simulink model "WindFarmType4AverageModel"  (R2024b)
settings: Solver=FixedStepDiscrete  StartTime=0.0  StopTime=5  RelTol=1e-4
PreLoadFcn:
  | Ts=50e-6;
InitFcn:
  | xInitial = WindFarmType4AverageModelInit;
  | Ts=50e-6;
undefined symbols (not defined in the file or in its folder): D1, D11, Delta, DiscIntNeverNeededParam, find_system
libraries: spsSecondOrderFilterLib x54, spsabctodq0Lib x30, spsThreePhaseVIMeasurementLib x26, simulink_extras x24, spsFirstOrderFilterLib x24, spsControlledVoltageSourceLib x18, spsThreePhaseTransformerTwoWindingsLib x14, spsThreePhasePISectionLineLib x14, simulink x12, spsSeriesRLCBranchLib x7, spsThreePhaseSeriesRLCLoadLib x7, spsSynchronousMachinepuStandardLib x7
(part 10 of 14)

== system WindFarmType4AverageModel/Noble Chateaugay (106.5 MW)/Wind Farm/Control/Grid-side converter Control system/INT ==
  note: INTEGRATOR (Trapezoidal) with External limits & Reset & Hold
  Max : Inport
  Min : Inport  Port=2
  In : Inport  Port=3
  Ki : Inport  Port=4
  Hold : Inport  Port=5
  Reset : Inport  Port=6
  Reset Value : Inport  Port=7
  Gain : Gain  Gain=Ts* 0.5  SaturateOnIntegerOverflow=on  OutDataTypeStr=Inherit: Same as input  ParamDataTypeStr=Inherit: Same as input
  IC = 0 : UnitDelay  SampleTime=Ts  HasFrameUpgradeWarning=on
  IC = i_ic : UnitDelay  SampleTime=Ts  HasFrameUpgradeWarning=on
  Logical Operator4 : Logic  Operator=OR
  MinMax : MinMax  Inputs=2  InputSameDT=on  SaturateOnIntegerOverflow=on
  MinMax1 : MinMax  Function=max  Inputs=2  InputSameDT=on  SaturateOnIntegerOverflow=on
  Product : Product  SaturateOnIntegerOverflow=on  OutDataTypeStr=Inherit: Same as first input
  S6 : Subsystem  mask(Limiter with External Limits){}
      mask Display: disp('      Limiter\n')
  Sum : Sum  InputSameDT=on  SaturateOnIntegerOverflow=on  OutDataTypeStr=Inherit: Same as first input
  Sum1 : Sum  InputSameDT=on  SaturateOnIntegerOverflow=on  OutDataTypeStr=Inherit: Same as first input
  Switch2 : Switch  Threshold=0.5
  Switch3 : Switch  Threshold=0.5
  Switch7 : Switch  Threshold=0.5
  Out : Outport  InitialOutput=0  VectorParamsAs1DForOutWhenUnconnected=off
  wires:
  Switch7/1 -> Switch3/1, Sum/2, Switch2/1
  IC = i_ic/1 -> Switch7/3
  Min/1 -> MinMax1/2, Switch3/3
  Switch3/1 -> MinMax1/1
  MinMax1/1 -> S6/3(MIN)
  MinMax/1 -> S6/1(MAX)
  Reset Value/1 -> Switch7/1
  Max/1 -> MinMax/2, Switch2/3
  Switch2/1 -> MinMax/1
  Logical Operator4/1 -> Switch3/2, Switch2/2
  Reset/1 -> Logical Operator4/2, Switch7/2
  Hold/1 -> Logical Operator4/1
  Sum/1 -> S6/2(In)
  Product/1 -> Sum/1
  In/1 -> Sum1/1, IC = 0/1
  IC = 0/1 -> Sum1/2
  Ki/1 -> Gain/1
  Sum1/1 -> Product/2
  Gain/1 -> Product/1
  S6/1("  ") -> Out/1, IC = i_ic/1

== system WindFarmType4AverageModel/Noble Chateaugay (106.5 MW)/Wind Farm/Control/Measurement and Transformation/Discrete 3-phase PLL-Driven Positive-Sequence Active & Reactive Power ==
  note: Pierre Giroux, Gilbert Sybille
      | Power System Simulation Laboratory
      | IREQ, Hydro-Quebc
  note: Discrete 3-phase PLL-driven Positive-Sequence Active & Reactive Power
  Freq : Inport  PortDimensions=1
  w : Inport  Port=2  PortDimensions=1
  Vabc : Inport  Port=3  PortDimensions=3
  Iabc : Inport  Port=4  PortDimensions=3
  Deg->Rad : Gain  Gain=pi/180  SaturateOnIntegerOverflow=on  OutDataTypeStr=Inherit: Same as input  ParamDataTypeStr=Inherit: Same as input
  Discrete 3-phase PLL-Driven Positive-Sequence Fundamental Value : Subsystem  mask(Discrete 3-phase PLL-Driven Positive-Sequence Fundamental Value){Finit=Finit, Fmin=Fmin, Par_Init=Par_Vinit, Ts=Ts}
      mask prompts: Finit "Initial frequency (Hz):"; Fmin "Minimum frequency (Hz):"; Par_Init "Initial input (positive component): [ Mag  Phase-relative-to-PLL(degrees) ]"; Ts "Sample time:"
      mask help:
      | For a supplied fundamental frequency (port Freq), this discrete block computes  the positive-sequence component (Magnitude and Phase)  of a set of three balanced or unbalanced signals (port abc) which may contain harmonics.
      |  Input port "Sin_Cos" (a two-dimension signal) provides the reference frame required for the computation..
      |  First and second outputs return respectively the magnitude and phase (in degrees relative to the PLL phase)) of the fundamental.
      | For the first cycle of simulation, the outputs are held constant to the values specified by the parameter "Initial input".
      | constant to the values specified by the parameter "Initial input". The value of the parameter "Minimum frequency" is used to determine the buffer size of the "Variable Transport Delay" block found inside this subsystem.
      mask init:
      | Real_Init=Par_Init(1)*cos(pi/180*Par_Init(2));
      | Imag_Init=Par_Init(1)*sin(pi/180*Par_Init(2));
      | power_initmask();
      settings: OpenFcn=power_openblockproxy();
  Discrete 3-phase PLL-Driven Positive-Sequence Fundamental Value2 : Subsystem  mask(Discrete 3-phase PLL-Driven Positive-Sequence Fundamental Value){Finit=Finit, Fmin=Fmin, Par_Init=Par_Iinit, Ts=Ts}
      mask prompts: Finit "Initial frequency (Hz):"; Fmin "Minimum frequency (Hz):"; Par_Init "Initial input (positive component): [ Mag  Phase-relative-to-PLL(degrees) ]"; Ts "Sample time:"
      mask help:
      | For a supplied fundamental frequency (port Freq), this discrete block computes  the positive-sequence component (Magnitude and Phase)  of a set of three balanced or unbalanced signals (port abc) which may contain harmonics.
      |  Input port "Sin_Cos" (a two-dimension signal) provides the reference frame required for the computation..
      |  First and second outputs return respectively the magnitude and phase (in degrees relative to the PLL phase)) of the fundamental.
      | For the first cycle of simulation, the outputs are held constant to the values specified by the parameter "Initial input".
      | constant to the values specified by the parameter "Initial input". The value of the parameter "Minimum frequency" is used to determine the buffer size of the "Variable Transport Delay" block found inside this subsystem.
      mask init:
      | Real_Init=Par_Init(1)*cos(pi/180*Par_Init(2));
      | Imag_Init=Par_Init(1)*sin(pi/180*Par_Init(2));
      | power_initmask();
      settings: OpenFcn=power_openblockproxy();
  Gain1 : Gain  Gain=3/2  SaturateOnIntegerOverflow=on  OutDataTypeStr=Inherit: Same as input  ParamDataTypeStr=Inherit: Same as input
  Mux2 : Mux  Inputs=2
  Mux3 : Mux  Inputs=2
  Product : Product  InputSameDT=on  SaturateOnIntegerOverflow=on  OutDataTypeStr=Inherit: Same as first input
  Product1 : Product  InputSameDT=on  SaturateOnIntegerOverflow=on  OutDataTypeStr=Inherit: Same as first input
  Product2 : Product  InputSameDT=on  SaturateOnIntegerOverflow=on  OutDataTypeStr=Inherit: Same as first input
  Sum : Sum  Inputs=+-  InputSameDT=on  SaturateOnIntegerOverflow=on  OutDataTypeStr=Inherit: Same as first input
  Trigonometric Function : Trigonometry
  Trigonometric Function1 : Trigonometry  Operator=cos
  Mag_V_I : Outport  VectorParamsAs1DForOutWhenUnconnected=off
  P_Q : Outport  Port=2  VectorParamsAs1DForOutWhenUnconnected=off
  wires:
  Iabc/1 -> Discrete 3-phase PLL-Driven Positive-Sequence Fundamental Value2/3(abc)
  Discrete 3-phase PLL-Driven Positive-Sequence Fundamental Value2/1(Mag) -> Product2/2, Mux3/2
  Product2/1 -> Product1/2, Product/1
  Gain1/1 -> P_Q/1
  Mux3/1 -> Mag_V_I/1
  Product1/1 -> Mux2/2
  Product/1 -> Mux2/1
  Mux2/1 -> Gain1/1
  Trigonometric Function/1 -> Product1/1
  Trigonometric Function1/1 -> Product/2
  Deg->Rad/1 -> Trigonometric Function/1, Trigonometric Function1/1
  Sum/1 -> Deg->Rad/1
  Discrete 3-phase PLL-Driven Positive-Sequence Fundamental Value2/2(Phase) -> Sum/2
  Discrete 3-phase PLL-Driven Positive-Sequence Fundamental Value/1(Mag) -> Product2/1, Mux3/1
  Discrete 3-phase PLL-Driven Positive-Sequence Fundamental Value/2(Phase) -> Sum/1
  w/1 -> Discrete 3-phase PLL-Driven Positive-Sequence Fundamental Value2/2(w), Discrete 3-phase PLL-Driven Positive-Sequence Fundamental Value/2(w)
  Freq/1 -> Discrete 3-phase PLL-Driven Positive-Sequence Fundamental Value2/1(Freq), Discrete 3-phase PLL-Driven Positive-Sequence Fundamental Value/1(Freq)
  Vabc/1 -> Discrete 3-phase PLL-Driven Positive-Sequence Fundamental Value/3(abc)

== system WindFarmType4AverageModel/Noble Chateaugay (106.5 MW)/Wind Farm/Control/Measurement and Transformation/Filter ==
  Vabc_grid : Inport
  Iabc_grid_conv : Inport  Port=2
  Vabc_LL_s : Inport  Port=3
  Iabc_stator : Inport  Port=4
  IL : Inport  Port=5
  Vdc : Inport  Port=6
  Qref : Inport  Port=7
  wr : Inport  Port=8
  angle_rotor : Inport  Port=9
  Second-Order Filter{,1..6} (7 alike) : spsSecondOrderFilterLib/Second-Order Filter  FilterType=Lowpass  Fo=Freq  Zeta=Zeta  Ts=Ts  Initialize=off  Vac_Init="[0,  0,  60]"  Vdc_Init=0  PlotResponse=off  FreqRange=[0, 500, 1]
  Second-Order Filter7 : spsSecondOrderFilterLib/Second-Order Filter  FilterType=Lowpass  Fo=Freq  Zeta=Zeta  Ts=Ts  Initialize=on  Vac_Init=[0.8 -25 60]*0  Vdc_Init=Vdc_nom  PlotResponse=off  FreqRange=[0, 500, 1]
  Second-Order Filter8 : spsSecondOrderFilterLib/Second-Order Filter  FilterType=Lowpass  Fo=Freq  Zeta=Zeta  Ts=Ts  Initialize=on  Vac_Init=[0.8 -25 60]*0  Vdc_Init=1+init(1)/100  PlotResponse=off  FreqRange=[0, 500, 1]
  "Vabc_grid " : Outport  VectorParamsAs1DForOutWhenUnconnected=off
  "Iabc_grid_conv " : Outport  Port=2  VectorParamsAs1DForOutWhenUnconnected=off
  "Vabc_LL_s " : Outport  Port=3  VectorParamsAs1DForOutWhenUnconnected=off
  "Iabc_stator " : Outport  Port=4  VectorParamsAs1DForOutWhenUnconnected=off
  "IL " : Outport  Port=5  VectorParamsAs1DForOutWhenUnconnected=off
  "Vdc " : Outport  Port=6  VectorParamsAs1DForOutWhenUnconnected=off
  "Qref " : Outport  Port=7  VectorParamsAs1DForOutWhenUnconnected=off
  "wr " : Outport  Port=8  VectorParamsAs1DForOutWhenUnconnected=off
  "angle_rotor " : Outport  Port=9  VectorParamsAs1DForOutWhenUnconnected=off
  wires:
  angle_rotor/1 -> Second-Order Filter6/1
  Second-Order Filter6/1 -> "angle_rotor "/1
  Second-Order Filter/1 -> "Vabc_grid "/1
  Second-Order Filter1/1 -> "Iabc_grid_conv "/1
  Vdc/1 -> Second-Order Filter7/1
  Second-Order Filter7/1 -> "Vdc "/1
  Second-Order Filter3/1 -> "Iabc_stator "/1
  wr/1 -> Second-Order Filter8/1
  Second-Order Filter8/1 -> "wr "/1
  Qref/1 -> Second-Order Filter5/1
  Second-Order Filter5/1 -> "Qref "/1
  IL/1 -> Second-Order Filter4/1
  Second-Order Filter4/1 -> "IL "/1
  Vabc_grid/1 -> Second-Order Filter/1
  Iabc_grid_conv/1 -> Second-Order Filter1/1
  Vabc_LL_s/1 -> Second-Order Filter2/1
  Second-Order Filter2/1 -> "Vabc_LL_s "/1
  Iabc_stator/1 -> Second-Order Filter3/1

== system WindFarmType4AverageModel/Noble Chateaugay (106.5 MW)/Wind Farm/Control/Measurement and Transformation/Stator flux estimator ==
  note: Quasi steady state flux at generator stator
  Vdqs : Inport
  Idqs : Inport  Port=2
  wr : Inport  Port=3
  Divide2 : Product  Inputs=**
  Divide4 : Product  Inputs=*/
  Divide7 : Product  Inputs=**
  Divide8 : Product  Inputs=*/
  First-Order Filter : spsFirstOrderFilterLib/First-Order Filter  FilterType=Lowpass  Tc=Flux_meas_time_constant  Ts=Ts  Initialize=on  Vac_Init=[0, 0, 0]  Vdc_Init=1  PlotResponse=off  FreqRange="[0,  200,  1]"
  Gain : Gain  Gain=-1
  Magnitude of flux : Fcn  Expr=sqrt(u(1)^2+u(2)^2)
  Mux1 : Mux  Inputs=2
  Rs2 : Constant  Value=Resistance
  Rs4 : Constant  Value=Resistance
  Selector1 : Selector  InputPortWidth=2  IndexOptions=Index vector (dialog)  Indices=2  OutputSizes=1
  Selector3 : Selector  InputPortWidth=2  IndexOptions=Index vector (dialog)  Indices=2  OutputSizes=1
  Selector7 : Selector  InputPortWidth=2  IndexOptions=Index vector (dialog)  Indices=1  OutputSizes=1
  Selector8 : Selector  InputPortWidth=2  IndexOptions=Index vector (dialog)  Indices=1  OutputSizes=1
  Sum2 : Sum  Inputs=|+-
  Sum4 : Sum  Inputs=|+-
  avoid division by 0 : Saturate  UpperLimit=inf  LowerLimit=1e-6
  Flux : Outport  VectorParamsAs1DForOutWhenUnconnected=off
  wires:
  First-Order Filter/1 -> Flux/1
  avoid division by 0/1 -> Gain/1, Divide4/2
  Magnitude of flux/1 -> First-Order Filter/1
  Mux1/1 -> Magnitude of flux/1
  Divide8/1 -> Mux1/2  "phi_q"
  Gain/1 -> Divide8/2
  Sum4/1 -> Divide8/1
  Selector8/1 -> Divide7/1  "Id"
  Rs4/1 -> Divide7/2
  Selector7/1 -> Sum4/1  "Vd"
  Divide7/1 -> Sum4/2  "Rs*Id"
  Idqs/1 -> Selector8/1, Selector3/1
  Vdqs/1 -> Selector7/1, Selector1/1
  Selector3/1 -> Divide2/1  "Iq"
  Rs2/1 -> Divide2/2
  Selector1/1 -> Sum2/1  "Vq"
  Divide2/1 -> Sum2/2  "Rs*Iq"
  Divide4/1 -> Mux1/1  "phi_d"
  Sum2/1 -> Divide4/1
  wr/1 -> avoid division by 0/1

== system WindFarmType4AverageModel/Noble Chateaugay (106.5 MW)/Wind Farm/Control/Measurement and Transformation/abc2qd ==
  note: This subsystem converts Vab and Vbc to Vd,Vq. The sine and cosine com-
      | puted here are sent to the inverse transformation subsystem qd/abc.
  Vabc_LL : Inport
  sin_cos : Inport  Port=2
  Fcn2 : Fcn  Expr=(u[4]*(2*u[1]+u[2]) + (sqrt(3)*u[2]*u[3])) * 1/3
  Fcn3 : Fcn  Expr=(u[3]*(2*u[1]+u[2]) + (-sqrt(3)*u[2]*u[4])) * 1/3
  Mux : Mux  Inputs=2
  Mux1 : Mux  Inputs=[ 2 2 ]
  Selector : Selector  InputPortWidth=3  IndexOptions=Index vector (dialog)  Indices=[1 2]  OutputSizes=1
  Vdq : Outport  InitialOutput=0  VectorParamsAs1DForOutWhenUnconnected=off
  wires:
  Fcn3/1 -> Mux/1
  Fcn2/1 -> Mux/2
  Mux1/1 -> Fcn3/1, Fcn2/1
  Vabc_LL/1 -> Selector/1
  sin_cos/1 -> Mux1/2
  Mux/1 -> Vdq/1
  Selector/1 -> Mux1/1

== system WindFarmType4AverageModel/Noble Chateaugay (106.5 MW)/Wind Farm/Control/Speed & Pitch Control/Discrete PI Controller ==
  note: Discrete PID Controller
  note: Pierre Giroux, Gilbert Sybille
      | Power System Simulation Laboratory
      | IREQ, Hydro-Quebc
  Error : Inport  SampleTime=Ts
  Discrete-Time Integrator : DiscreteIntegrator  InitialCondition=Init  SampleTime=Ts  LimitOutput=on  UpperSaturationLimit=UpperLimit  LowerSaturationLimit=LowerLimit  ICPrevOutput=DiscIntNeverNeededParam  ICPrevScaledInput=DiscIntNeverNeededParam
  Kp4 : Gain  Gain=Kp  SaturateOnIntegerOverflow=on  SampleTime=Ts  OutDataTypeStr=Inherit: Same as input  ParamDataTypeStr=Inherit: Same as input
  Kp5 : Gain  Gain=Ki  SaturateOnIntegerOverflow=on  SampleTime=Ts  OutDataTypeStr=Inherit: Same as input  ParamDataTypeStr=Inherit: Same as input
  Saturation2 : Saturate  UpperLimit=UpperLimit  LowerLimit=LowerLimit  SampleTime=Ts
  Sum6 : Sum  InputSameDT=on  SaturateOnIntegerOverflow=on  SampleTime=Ts  OutDataTypeStr=Inherit: Same as first input
  Zero-Order Hold : ZeroOrderHold  SampleTime=Ts
  Out : Outport  SampleTime=Ts  InitialOutput=0  VectorParamsAs1DForOutWhenUnconnected=off
  wires:
  Zero-Order Hold/1 -> Sum6/1
  Saturation2/1 -> Out/1
  Discrete-Time Integrator/1 -> Sum6/2
  Kp4/1 -> Zero-Order Hold/1
  Kp5/1 -> Discrete-Time Integrator/1
  Sum6/1 -> Saturation2/1
  Error/1 -> Kp5/1, Kp4/1

== system WindFarmType4AverageModel/Noble Chateaugay (106.5 MW)/Wind Farm/Control/Speed & Pitch Control/Discrete PI Controller1 ==
  note: Discrete PID Controller
  note: Pierre Giroux, Gilbert Sybille
      | Power System Simulation Laboratory
      | IREQ, Hydro-Quebc
  Error : Inport  SampleTime=Ts
  Discrete-Time Integrator : DiscreteIntegrator  InitialCondition=Init  SampleTime=Ts  LimitOutput=on  UpperSaturationLimit=UpperLimit  LowerSaturationLimit=LowerLimit  ICPrevOutput=DiscIntNeverNeededParam  ICPrevScaledInput=DiscIntNeverNeededParam
  Kp4 : Gain  Gain=Kp  SaturateOnIntegerOverflow=on  SampleTime=Ts  OutDataTypeStr=Inherit: Same as input  ParamDataTypeStr=Inherit: Same as input
  Kp5 : Gain  Gain=Ki  SaturateOnIntegerOverflow=on  SampleTime=Ts  OutDataTypeStr=Inherit: Same as input  ParamDataTypeStr=Inherit: Same as input
  Saturation2 : Saturate  UpperLimit=UpperLimit  LowerLimit=LowerLimit  SampleTime=Ts
  Sum6 : Sum  InputSameDT=on  SaturateOnIntegerOverflow=on  SampleTime=Ts  OutDataTypeStr=Inherit: Same as first input
  Zero-Order Hold : ZeroOrderHold  SampleTime=Ts
  Out : Outport  SampleTime=Ts  InitialOutput=0  VectorParamsAs1DForOutWhenUnconnected=off
  wires:
  Zero-Order Hold/1 -> Sum6/1
  Saturation2/1 -> Out/1
  Discrete-Time Integrator/1 -> Sum6/2
  Kp4/1 -> Zero-Order Hold/1
  Kp5/1 -> Discrete-Time Integrator/1
  Sum6/1 -> Saturation2/1
  Error/1 -> Kp5/1, Kp4/1

== system WindFarmType4AverageModel/Noble Chateaugay (106.5 MW)/Wind Farm/Control/Speed & Pitch Control/Discrete PI Controller2 ==
  note: Discrete PID Controller
  note: Pierre Giroux, Gilbert Sybille
      | Power System Simulation Laboratory
      | IREQ, Hydro-Quebc
  Error : Inport  SampleTime=Ts
  Discrete-Time Integrator : DiscreteIntegrator  InitialCondition=Init  SampleTime=Ts  LimitOutput=on  UpperSaturationLimit=UpperLimit  LowerSaturationLimit=LowerLimit  ICPrevOutput=DiscIntNeverNeededParam  ICPrevScaledInput=DiscIntNeverNeededParam
  Kp4 : Gain  Gain=Kp  SaturateOnIntegerOverflow=on  SampleTime=Ts  OutDataTypeStr=Inherit: Same as input  ParamDataTypeStr=Inherit: Same as input
  Kp5 : Gain  Gain=Ki  SaturateOnIntegerOverflow=on  SampleTime=Ts  OutDataTypeStr=Inherit: Same as input  ParamDataTypeStr=Inherit: Same as input
  Saturation2 : Saturate  UpperLimit=UpperLimit  LowerLimit=LowerLimit  SampleTime=Ts
  Sum6 : Sum  InputSameDT=on  SaturateOnIntegerOverflow=on  SampleTime=Ts  OutDataTypeStr=Inherit: Same as first input
  Zero-Order Hold : ZeroOrderHold  SampleTime=Ts
  Out : Outport  SampleTime=Ts  InitialOutput=0  VectorParamsAs1DForOutWhenUnconnected=off
  wires:
  Zero-Order Hold/1 -> Sum6/1
  Saturation2/1 -> Out/1
  Discrete-Time Integrator/1 -> Sum6/2
  Kp4/1 -> Zero-Order Hold/1
  Kp5/1 -> Discrete-Time Integrator/1
  Sum6/1 -> Saturation2/1
  Error/1 -> Kp5/1, Kp4/1

== system WindFarmType4AverageModel/Noble Clinton (100.5 MW)/Wind Farm/Control/Excitation Control system/Discrete PI Controller ==
  note: Discrete PID Controller
  note: Pierre Giroux, Gilbert Sybille
      | Power System Simulation Laboratory
      | IREQ, Hydro-Quebc
  Error : Inport  SampleTime=Ts
  Discrete-Time Integrator : DiscreteIntegrator  InitialCondition=Init  SampleTime=Ts  LimitOutput=on  UpperSaturationLimit=UpperLimit  LowerSaturationLimit=LowerLimit  ICPrevOutput=DiscIntNeverNeededParam  ICPrevScaledInput=DiscIntNeverNeededParam
  Kp4 : Gain  Gain=Kp  SaturateOnIntegerOverflow=on  SampleTime=Ts  OutDataTypeStr=Inherit: Same as input  ParamDataTypeStr=Inherit: Same as input
  Kp5 : Gain  Gain=Ki  SaturateOnIntegerOverflow=on  SampleTime=Ts  OutDataTypeStr=Inherit: Same as input  ParamDataTypeStr=Inherit: Same as input
  Saturation2 : Saturate  UpperLimit=UpperLimit  LowerLimit=LowerLimit  SampleTime=Ts
  Sum6 : Sum  InputSameDT=on  SaturateOnIntegerOverflow=on  SampleTime=Ts  OutDataTypeStr=Inherit: Same as first input
  Zero-Order Hold : ZeroOrderHold  SampleTime=Ts
  Out : Outport  SampleTime=Ts  InitialOutput=0  VectorParamsAs1DForOutWhenUnconnected=off
  wires:
  Zero-Order Hold/1 -> Sum6/1
  Saturation2/1 -> Out/1
  Discrete-Time Integrator/1 -> Sum6/2
  Kp4/1 -> Zero-Order Hold/1
  Kp5/1 -> Discrete-Time Integrator/1
  Sum6/1 -> Saturation2/1
  Error/1 -> Kp5/1, Kp4/1

== system WindFarmType4AverageModel/Noble Clinton (100.5 MW)/Wind Farm/Control/Grid-side converter Control system/Discrete PI Controller ==
  note: Discrete PID Controller
  note: Pierre Giroux, Gilbert Sybille
      | Power System Simulation Laboratory
      | IREQ, Hydro-Quebc
  Error : Inport  SampleTime=Ts
  Discrete-Time Integrator : DiscreteIntegrator  InitialCondition=Init  SampleTime=Ts  LimitOutput=on  UpperSaturationLimit=UpperLimit  LowerSaturationLimit=LowerLimit  ICPrevOutput=DiscIntNeverNeededParam  ICPrevScaledInput=DiscIntNeverNeededParam
  Kp4 : Gain  Gain=Kp  SaturateOnIntegerOverflow=on  SampleTime=Ts  OutDataTypeStr=Inherit: Same as input  ParamDataTypeStr=Inherit: Same as input
  Kp5 : Gain  Gain=Ki  SaturateOnIntegerOverflow=on  SampleTime=Ts  OutDataTypeStr=Inherit: Same as input  ParamDataTypeStr=Inherit: Same as input
  Saturation2 : Saturate  UpperLimit=UpperLimit  LowerLimit=LowerLimit  SampleTime=Ts
  Sum6 : Sum  InputSameDT=on  SaturateOnIntegerOverflow=on  SampleTime=Ts  OutDataTypeStr=Inherit: Same as first input
  Zero-Order Hold : ZeroOrderHold  SampleTime=Ts
  Out : Outport  SampleTime=Ts  InitialOutput=0  VectorParamsAs1DForOutWhenUnconnected=off
  wires:
  Zero-Order Hold/1 -> Sum6/1
  Saturation2/1 -> Out/1
  Discrete-Time Integrator/1 -> Sum6/2
  Kp4/1 -> Zero-Order Hold/1
  Kp5/1 -> Discrete-Time Integrator/1
  Sum6/1 -> Saturation2/1
  Error/1 -> Kp5/1, Kp4/1

== system WindFarmType4AverageModel/Noble Clinton (100.5 MW)/Wind Farm/Control/Grid-side converter Control system/Discrete PI Controller1 ==
  note: Discrete PID Controller
  note: Pierre Giroux, Gilbert Sybille
      | Power System Simulation Laboratory
      | IREQ, Hydro-Quebc
  Error : Inport  SampleTime=Ts
  Discrete-Time Integrator : DiscreteIntegrator  InitialCondition=Init  SampleTime=Ts  LimitOutput=on  UpperSaturationLimit=UpperLimit  LowerSaturationLimit=LowerLimit  ICPrevOutput=DiscIntNeverNeededParam  ICPrevScaledInput=DiscIntNeverNeededParam
  Kp4 : Gain  Gain=Kp  SaturateOnIntegerOverflow=on  SampleTime=Ts  OutDataTypeStr=Inherit: Same as input  ParamDataTypeStr=Inherit: Same as input
  Kp5 : Gain  Gain=Ki  SaturateOnIntegerOverflow=on  SampleTime=Ts  OutDataTypeStr=Inherit: Same as input  ParamDataTypeStr=Inherit: Same as input
  Saturation2 : Saturate  UpperLimit=UpperLimit  LowerLimit=LowerLimit  SampleTime=Ts
  Sum6 : Sum  InputSameDT=on  SaturateOnIntegerOverflow=on  SampleTime=Ts  OutDataTypeStr=Inherit: Same as first input
  Zero-Order Hold : ZeroOrderHold  SampleTime=Ts
  Out : Outport  SampleTime=Ts  InitialOutput=0  VectorParamsAs1DForOutWhenUnconnected=off
  wires:
  Zero-Order Hold/1 -> Sum6/1
  Saturation2/1 -> Out/1
  Discrete-Time Integrator/1 -> Sum6/2
  Kp4/1 -> Zero-Order Hold/1
  Kp5/1 -> Discrete-Time Integrator/1
  Sum6/1 -> Saturation2/1
  Error/1 -> Kp5/1, Kp4/1

== system WindFarmType4AverageModel/Noble Clinton (100.5 MW)/Wind Farm/Control/Grid-side converter Control system/INT ==
  note: INTEGRATOR (Trapezoidal) with External limits & Reset & Hold
  Max : Inport
  Min : Inport  Port=2
  In : Inport  Port=3
  Ki : Inport  Port=4
  Hold : Inport  Port=5
  Reset : Inport  Port=6
  Reset Value : Inport  Port=7
  Gain : Gain  Gain=Ts* 0.5  SaturateOnIntegerOverflow=on  OutDataTypeStr=Inherit: Same as input  ParamDataTypeStr=Inherit: Same as input
  IC = 0 : UnitDelay  SampleTime=Ts  HasFrameUpgradeWarning=on
  IC = i_ic : UnitDelay  SampleTime=Ts  HasFrameUpgradeWarning=on
  Logical Operator4 : Logic  Operator=OR
  MinMax : MinMax  Inputs=2  InputSameDT=on  SaturateOnIntegerOverflow=on
  MinMax1 : MinMax  Function=max  Inputs=2  InputSameDT=on  SaturateOnIntegerOverflow=on
  Product : Product  SaturateOnIntegerOverflow=on  OutDataTypeStr=Inherit: Same as first input
  S6 : Subsystem  mask(Limiter with External Limits){}
      mask Display: disp('      Limiter\n')
  Sum : Sum  InputSameDT=on  SaturateOnIntegerOverflow=on  OutDataTypeStr=Inherit: Same as first input
  Sum1 : Sum  InputSameDT=on  SaturateOnIntegerOverflow=on  OutDataTypeStr=Inherit: Same as first input
  Switch2 : Switch  Threshold=0.5
  Switch3 : Switch  Threshold=0.5
  Switch7 : Switch  Threshold=0.5
  Out : Outport  InitialOutput=0  VectorParamsAs1DForOutWhenUnconnected=off
  wires:
  Switch7/1 -> Switch3/1, Sum/2, Switch2/1
  IC = i_ic/1 -> Switch7/3
  Min/1 -> MinMax1/2, Switch3/3
  Switch3/1 -> MinMax1/1
  MinMax1/1 -> S6/3(MIN)
  MinMax/1 -> S6/1(MAX)
  Reset Value/1 -> Switch7/1
  Max/1 -> MinMax/2, Switch2/3
  Switch2/1 -> MinMax/1
  Logical Operator4/1 -> Switch3/2, Switch2/2
  Reset/1 -> Logical Operator4/2, Switch7/2
  Hold/1 -> Logical Operator4/1
  Sum/1 -> S6/2(In)
  Product/1 -> Sum/1
  In/1 -> Sum1/1, IC = 0/1
  IC = 0/1 -> Sum1/2
  Ki/1 -> Gain/1
  Sum1/1 -> Product/2
  Gain/1 -> Product/1
  S6/1("  ") -> Out/1, IC = i_ic/1

== system WindFarmType4AverageModel/Noble Clinton (100.5 MW)/Wind Farm/Control/Measurement and Transformation/Discrete 3-phase PLL-Driven Positive-Sequence Active & Reactive Power ==
  note: Pierre Giroux, Gilbert Sybille
      | Power System Simulation Laboratory
      | IREQ, Hydro-Quebc
  note: Discrete 3-phase PLL-driven Positive-Sequence Active & Reactive Power
  Freq : Inport  PortDimensions=1
  w : Inport  Port=2  PortDimensions=1
  Vabc : Inport  Port=3  PortDimensions=3
  Iabc : Inport  Port=4  PortDimensions=3
  Deg->Rad : Gain  Gain=pi/180  SaturateOnIntegerOverflow=on  OutDataTypeStr=Inherit: Same as input  ParamDataTypeStr=Inherit: Same as input
  Discrete 3-phase PLL-Driven Positive-Sequence Fundamental Value : Subsystem  mask(Discrete 3-phase PLL-Driven Positive-Sequence Fundamental Value){Finit=Finit, Fmin=Fmin, Par_Init=Par_Vinit, Ts=Ts}
      mask prompts: Finit "Initial frequency (Hz):"; Fmin "Minimum frequency (Hz):"; Par_Init "Initial input (positive component): [ Mag  Phase-relative-to-PLL(degrees) ]"; Ts "Sample time:"
      mask help:
      | For a supplied fundamental frequency (port Freq), this discrete block computes  the positive-sequence component (Magnitude and Phase)  of a set of three balanced or unbalanced signals (port abc) which may contain harmonics.
      |  Input port "Sin_Cos" (a two-dimension signal) provides the reference frame required for the computation..
      |  First and second outputs return respectively the magnitude and phase (in degrees relative to the PLL phase)) of the fundamental.
      | For the first cycle of simulation, the outputs are held constant to the values specified by the parameter "Initial input".
      | constant to the values specified by the parameter "Initial input". The value of the parameter "Minimum frequency" is used to determine the buffer size of the "Variable Transport Delay" block found inside this subsystem.
      mask init:
      | Real_Init=Par_Init(1)*cos(pi/180*Par_Init(2));
      | Imag_Init=Par_Init(1)*sin(pi/180*Par_Init(2));
      | power_initmask();
      settings: OpenFcn=power_openblockproxy();
  Discrete 3-phase PLL-Driven Positive-Sequence Fundamental Value2 : Subsystem  mask(Discrete 3-phase PLL-Driven Positive-Sequence Fundamental Value){Finit=Finit, Fmin=Fmin, Par_Init=Par_Iinit, Ts=Ts}
      mask prompts: Finit "Initial frequency (Hz):"; Fmin "Minimum frequency (Hz):"; Par_Init "Initial input (positive component): [ Mag  Phase-relative-to-PLL(degrees) ]"; Ts "Sample time:"
      mask help:
      | For a supplied fundamental frequency (port Freq), this discrete block computes  the positive-sequence component (Magnitude and Phase)  of a set of three balanced or unbalanced signals (port abc) which may contain harmonics.
      |  Input port "Sin_Cos" (a two-dimension signal) provides the reference frame required for the computation..
      |  First and second outputs return respectively the magnitude and phase (in degrees relative to the PLL phase)) of the fundamental.
      | For the first cycle of simulation, the outputs are held constant to the values specified by the parameter "Initial input".
      | constant to the values specified by the parameter "Initial input". The value of the parameter "Minimum frequency" is used to determine the buffer size of the "Variable Transport Delay" block found inside this subsystem.
      mask init:
      | Real_Init=Par_Init(1)*cos(pi/180*Par_Init(2));
      | Imag_Init=Par_Init(1)*sin(pi/180*Par_Init(2));
      | power_initmask();
      settings: OpenFcn=power_openblockproxy();
  Gain1 : Gain  Gain=3/2  SaturateOnIntegerOverflow=on  OutDataTypeStr=Inherit: Same as input  ParamDataTypeStr=Inherit: Same as input
  Mux2 : Mux  Inputs=2
  Mux3 : Mux  Inputs=2
  Product : Product  InputSameDT=on  SaturateOnIntegerOverflow=on  OutDataTypeStr=Inherit: Same as first input
  Product1 : Product  InputSameDT=on  SaturateOnIntegerOverflow=on  OutDataTypeStr=Inherit: Same as first input
  Product2 : Product  InputSameDT=on  SaturateOnIntegerOverflow=on  OutDataTypeStr=Inherit: Same as first input
  Sum : Sum  Inputs=+-  InputSameDT=on  SaturateOnIntegerOverflow=on  OutDataTypeStr=Inherit: Same as first input
  Trigonometric Function : Trigonometry
  Trigonometric Function1 : Trigonometry  Operator=cos
  Mag_V_I : Outport  VectorParamsAs1DForOutWhenUnconnected=off
  P_Q : Outport  Port=2  VectorParamsAs1DForOutWhenUnconnected=off
  wires:
  Iabc/1 -> Discrete 3-phase PLL-Driven Positive-Sequence Fundamental Value2/3(abc)
  Discrete 3-phase PLL-Driven Positive-Sequence Fundamental Value2/1(Mag) -> Product2/2, Mux3/2
  Product2/1 -> Product1/2, Product/1
  Gain1/1 -> P_Q/1
  Mux3/1 -> Mag_V_I/1
  Product1/1 -> Mux2/2
  Product/1 -> Mux2/1
  Mux2/1 -> Gain1/1
  Trigonometric Function/1 -> Product1/1
  Trigonometric Function1/1 -> Product/2
  Deg->Rad/1 -> Trigonometric Function/1, Trigonometric Function1/1
  Sum/1 -> Deg->Rad/1
  Discrete 3-phase PLL-Driven Positive-Sequence Fundamental Value2/2(Phase) -> Sum/2
  Discrete 3-phase PLL-Driven Positive-Sequence Fundamental Value/1(Mag) -> Product2/1, Mux3/1
  Discrete 3-phase PLL-Driven Positive-Sequence Fundamental Value/2(Phase) -> Sum/1
  w/1 -> Discrete 3-phase PLL-Driven Positive-Sequence Fundamental Value2/2(w), Discrete 3-phase PLL-Driven Positive-Sequence Fundamental Value/2(w)
  Freq/1 -> Discrete 3-phase PLL-Driven Positive-Sequence Fundamental Value2/1(Freq), Discrete 3-phase PLL-Driven Positive-Sequence Fundamental Value/1(Freq)
  Vabc/1 -> Discrete 3-phase PLL-Driven Positive-Sequence Fundamental Value/3(abc)

== system WindFarmType4AverageModel/Noble Clinton (100.5 MW)/Wind Farm/Control/Measurement and Transformation/Filter ==
  Vabc_grid : Inport
  Iabc_grid_conv : Inport  Port=2
  Vabc_LL_s : Inport  Port=3
  Iabc_stator : Inport  Port=4
  IL : Inport  Port=5
  Vdc : Inport  Port=6
  Qref : Inport  Port=7
  wr : Inport  Port=8
  angle_rotor : Inport  Port=9
  Second-Order Filter{,1..6} (7 alike) : spsSecondOrderFilterLib/Second-Order Filter  FilterType=Lowpass  Fo=Freq  Zeta=Zeta  Ts=Ts  Initialize=off  Vac_Init="[0,  0,  60]"  Vdc_Init=0  PlotResponse=off  FreqRange=[0, 500, 1]
  Second-Order Filter7 : spsSecondOrderFilterLib/Second-Order Filter  FilterType=Lowpass  Fo=Freq  Zeta=Zeta  Ts=Ts  Initialize=on  Vac_Init=[0.8 -25 60]*0  Vdc_Init=Vdc_nom  PlotResponse=off  FreqRange=[0, 500, 1]
  Second-Order Filter8 : spsSecondOrderFilterLib/Second-Order Filter  FilterType=Lowpass  Fo=Freq  Zeta=Zeta  Ts=Ts  Initialize=on  Vac_Init=[0.8 -25 60]*0  Vdc_Init=1+init(1)/100  PlotResponse=off  FreqRange=[0, 500, 1]
  "Vabc_grid " : Outport  VectorParamsAs1DForOutWhenUnconnected=off
  "Iabc_grid_conv " : Outport  Port=2  VectorParamsAs1DForOutWhenUnconnected=off
  "Vabc_LL_s " : Outport  Port=3  VectorParamsAs1DForOutWhenUnconnected=off
  "Iabc_stator " : Outport  Port=4  VectorParamsAs1DForOutWhenUnconnected=off
  "IL " : Outport  Port=5  VectorParamsAs1DForOutWhenUnconnected=off
  "Vdc " : Outport  Port=6  VectorParamsAs1DForOutWhenUnconnected=off
  "Qref " : Outport  Port=7  VectorParamsAs1DForOutWhenUnconnected=off
  "wr " : Outport  Port=8  VectorParamsAs1DForOutWhenUnconnected=off
  "angle_rotor " : Outport  Port=9  VectorParamsAs1DForOutWhenUnconnected=off
  wires:
  angle_rotor/1 -> Second-Order Filter6/1
  Second-Order Filter6/1 -> "angle_rotor "/1
  Second-Order Filter/1 -> "Vabc_grid "/1
  Second-Order Filter1/1 -> "Iabc_grid_conv "/1
  Vdc/1 -> Second-Order Filter7/1
  Second-Order Filter7/1 -> "Vdc "/1
  Second-Order Filter3/1 -> "Iabc_stator "/1
  wr/1 -> Second-Order Filter8/1
  Second-Order Filter8/1 -> "wr "/1
  Qref/1 -> Second-Order Filter5/1
  Second-Order Filter5/1 -> "Qref "/1
  IL/1 -> Second-Order Filter4/1
  Second-Order Filter4/1 -> "IL "/1
  Vabc_grid/1 -> Second-Order Filter/1
  Iabc_grid_conv/1 -> Second-Order Filter1/1
  Vabc_LL_s/1 -> Second-Order Filter2/1
  Second-Order Filter2/1 -> "Vabc_LL_s "/1
  Iabc_stator/1 -> Second-Order Filter3/1

== system WindFarmType4AverageModel/Noble Clinton (100.5 MW)/Wind Farm/Control/Measurement and Transformation/Stator flux estimator ==
  note: Quasi steady state flux at generator stator
  Vdqs : Inport
  Idqs : Inport  Port=2
  wr : Inport  Port=3
  Divide2 : Product  Inputs=**
  Divide4 : Product  Inputs=*/
  Divide7 : Product  Inputs=**
  Divide8 : Product  Inputs=*/
  First-Order Filter : spsFirstOrderFilterLib/First-Order Filter  FilterType=Lowpass  Tc=Flux_meas_time_constant  Ts=Ts  Initialize=on  Vac_Init=[0, 0, 0]  Vdc_Init=1  PlotResponse=off  FreqRange="[0,  200,  1]"
  Gain : Gain  Gain=-1
  Magnitude of flux : Fcn  Expr=sqrt(u(1)^2+u(2)^2)
  Mux1 : Mux  Inputs=2
  Rs2 : Constant  Value=Resistance
  Rs4 : Constant  Value=Resistance
  Selector1 : Selector  InputPortWidth=2  IndexOptions=Index vector (dialog)  Indices=2  OutputSizes=1
  Selector3 : Selector  InputPortWidth=2  IndexOptions=Index vector (dialog)  Indices=2  OutputSizes=1
  Selector7 : Selector  InputPortWidth=2  IndexOptions=Index vector (dialog)  Indices=1  OutputSizes=1
  Selector8 : Selector  InputPortWidth=2  IndexOptions=Index vector (dialog)  Indices=1  OutputSizes=1
  Sum2 : Sum  Inputs=|+-
  Sum4 : Sum  Inputs=|+-
  avoid division by 0 : Saturate  UpperLimit=inf  LowerLimit=1e-6
  Flux : Outport  VectorParamsAs1DForOutWhenUnconnected=off
  wires:
  First-Order Filter/1 -> Flux/1
  avoid division by 0/1 -> Gain/1, Divide4/2
  Magnitude of flux/1 -> First-Order Filter/1
  Mux1/1 -> Magnitude of flux/1
  Divide8/1 -> Mux1/2  "phi_q"
  Gain/1 -> Divide8/2
  Sum4/1 -> Divide8/1
  Selector8/1 -> Divide7/1  "Id"
  Rs4/1 -> Divide7/2
  Selector7/1 -> Sum4/1  "Vd"
  Divide7/1 -> Sum4/2  "Rs*Id"
  Idqs/1 -> Selector8/1, Selector3/1
  Vdqs/1 -> Selector7/1, Selector1/1
  Selector3/1 -> Divide2/1  "Iq"
  Rs2/1 -> Divide2/2
  Selector1/1 -> Sum2/1  "Vq"
  Divide2/1 -> Sum2/2  "Rs*Iq"
  Divide4/1 -> Mux1/1  "phi_d"
  Sum2/1 -> Divide4/1
  wr/1 -> avoid division by 0/1

== system WindFarmType4AverageModel/Noble Clinton (100.5 MW)/Wind Farm/Control/Measurement and Transformation/abc2qd ==
  note: This subsystem converts Vab and Vbc to Vd,Vq. The sine and cosine com-
      | puted here are sent to the inverse transformation subsystem qd/abc.
  Vabc_LL : Inport
  sin_cos : Inport  Port=2
  Fcn2 : Fcn  Expr=(u[4]*(2*u[1]+u[2]) + (sqrt(3)*u[2]*u[3])) * 1/3
  Fcn3 : Fcn  Expr=(u[3]*(2*u[1]+u[2]) + (-sqrt(3)*u[2]*u[4])) * 1/3
  Mux : Mux  Inputs=2
  Mux1 : Mux  Inputs=[ 2 2 ]
  Selector : Selector  InputPortWidth=3  IndexOptions=Index vector (dialog)  Indices=[1 2]  OutputSizes=1
  Vdq : Outport  InitialOutput=0  VectorParamsAs1DForOutWhenUnconnected=off
  wires:
  Fcn3/1 -> Mux/1
  Fcn2/1 -> Mux/2
  Mux1/1 -> Fcn3/1, Fcn2/1
  Vabc_LL/1 -> Selector/1
  sin_cos/1 -> Mux1/2
  Mux/1 -> Vdq/1
  Selector/1 -> Mux1/1

== system WindFarmType4AverageModel/Noble Clinton (100.5 MW)/Wind Farm/Control/Speed & Pitch Control/Discrete PI Controller ==
  note: Discrete PID Controller
  note: Pierre Giroux, Gilbert Sybille
      | Power System Simulation Laboratory
      | IREQ, Hydro-Quebc
  Error : Inport  SampleTime=Ts
  Discrete-Time Integrator : DiscreteIntegrator  InitialCondition=Init  SampleTime=Ts  LimitOutput=on  UpperSaturationLimit=UpperLimit  LowerSaturationLimit=LowerLimit  ICPrevOutput=DiscIntNeverNeededParam  ICPrevScaledInput=DiscIntNeverNeededParam
  Kp4 : Gain  Gain=Kp  SaturateOnIntegerOverflow=on  SampleTime=Ts  OutDataTypeStr=Inherit: Same as input  ParamDataTypeStr=Inherit: Same as input
  Kp5 : Gain  Gain=Ki  SaturateOnIntegerOverflow=on  SampleTime=Ts  OutDataTypeStr=Inherit: Same as input  ParamDataTypeStr=Inherit: Same as input
  Saturation2 : Saturate  UpperLimit=UpperLimit  LowerLimit=LowerLimit  SampleTime=Ts
  Sum6 : Sum  InputSameDT=on  SaturateOnIntegerOverflow=on  SampleTime=Ts  OutDataTypeStr=Inherit: Same as first input
  Zero-Order Hold : ZeroOrderHold  SampleTime=Ts
  Out : Outport  SampleTime=Ts  InitialOutput=0  VectorParamsAs1DForOutWhenUnconnected=off
  wires:
  Zero-Order Hold/1 -> Sum6/1
  Saturation2/1 -> Out/1
  Discrete-Time Integrator/1 -> Sum6/2
  Kp4/1 -> Zero-Order Hold/1
  Kp5/1 -> Discrete-Time Integrator/1
  Sum6/1 -> Saturation2/1
  Error/1 -> Kp5/1, Kp4/1

== system WindFarmType4AverageModel/Noble Clinton (100.5 MW)/Wind Farm/Control/Speed & Pitch Control/Discrete PI Controller1 ==
  note: Discrete PID Controller
  note: Pierre Giroux, Gilbert Sybille
      | Power System Simulation Laboratory
      | IREQ, Hydro-Quebc
  Error : Inport  SampleTime=Ts
  Discrete-Time Integrator : DiscreteIntegrator  InitialCondition=Init  SampleTime=Ts  LimitOutput=on  UpperSaturationLimit=UpperLimit  LowerSaturationLimit=LowerLimit  ICPrevOutput=DiscIntNeverNeededParam  ICPrevScaledInput=DiscIntNeverNeededParam
  Kp4 : Gain  Gain=Kp  SaturateOnIntegerOverflow=on  SampleTime=Ts  OutDataTypeStr=Inherit: Same as input  ParamDataTypeStr=Inherit: Same as input
  Kp5 : Gain  Gain=Ki  SaturateOnIntegerOverflow=on  SampleTime=Ts  OutDataTypeStr=Inherit: Same as input  ParamDataTypeStr=Inherit: Same as input
  Saturation2 : Saturate  UpperLimit=UpperLimit  LowerLimit=LowerLimit  SampleTime=Ts
  Sum6 : Sum  InputSameDT=on  SaturateOnIntegerOverflow=on  SampleTime=Ts  OutDataTypeStr=Inherit: Same as first input
  Zero-Order Hold : ZeroOrderHold  SampleTime=Ts
  Out : Outport  SampleTime=Ts  InitialOutput=0  VectorParamsAs1DForOutWhenUnconnected=off
  wires:
  Zero-Order Hold/1 -> Sum6/1
  Saturation2/1 -> Out/1
  Discrete-Time Integrator/1 -> Sum6/2
  Kp4/1 -> Zero-Order Hold/1
  Kp5/1 -> Discrete-Time Integrator/1
  Sum6/1 -> Saturation2/1
  Error/1 -> Kp5/1, Kp4/1

== system WindFarmType4AverageModel/Noble Clinton (100.5 MW)/Wind Farm/Control/Speed & Pitch Control/Discrete PI Controller2 ==
  note: Discrete PID Controller
  note: Pierre Giroux, Gilbert Sybille
      | Power System Simulation Laboratory
      | IREQ, Hydro-Quebc
  Error : Inport  SampleTime=Ts
  Discrete-Time Integrator : DiscreteIntegrator  InitialCondition=Init  SampleTime=Ts  LimitOutput=on  UpperSaturationLimit=UpperLimit  LowerSaturationLimit=LowerLimit  ICPrevOutput=DiscIntNeverNeededParam  ICPrevScaledInput=DiscIntNeverNeededParam
  Kp4 : Gain  Gain=Kp  SaturateOnIntegerOverflow=on  SampleTime=Ts  OutDataTypeStr=Inherit: Same as input  ParamDataTypeStr=Inherit: Same as input
  Kp5 : Gain  Gain=Ki  SaturateOnIntegerOverflow=on  SampleTime=Ts  OutDataTypeStr=Inherit: Same as input  ParamDataTypeStr=Inherit: Same as input
  Saturation2 : Saturate  UpperLimit=UpperLimit  LowerLimit=LowerLimit  SampleTime=Ts
  Sum6 : Sum  InputSameDT=on  SaturateOnIntegerOverflow=on  SampleTime=Ts  OutDataTypeStr=Inherit: Same as first input
  Zero-Order Hold : ZeroOrderHold  SampleTime=Ts
  Out : Outport  SampleTime=Ts  InitialOutput=0  VectorParamsAs1DForOutWhenUnconnected=off
  wires:
  Zero-Order Hold/1 -> Sum6/1
  Saturation2/1 -> Out/1
  Discrete-Time Integrator/1 -> Sum6/2
  Kp4/1 -> Zero-Order Hold/1
  Kp5/1 -> Discrete-Time Integrator/1
  Sum6/1 -> Saturation2/1
  Error/1 -> Kp5/1, Kp4/1

== system WindFarmType4AverageModel/Noble Ellenburg (81 MW)/Wind Farm/Control/Excitation Control system/Discrete PI Controller ==
  note: Discrete PID Controller
  note: Pierre Giroux, Gilbert Sybille
      | Power System Simulation Laboratory
      | IREQ, Hydro-Quebc
  Error : Inport  SampleTime=Ts
  Discrete-Time Integrator : DiscreteIntegrator  InitialCondition=Init  SampleTime=Ts  LimitOutput=on  UpperSaturationLimit=UpperLimit  LowerSaturationLimit=LowerLimit  ICPrevOutput=DiscIntNeverNeededParam  ICPrevScaledInput=DiscIntNeverNeededParam
  Kp4 : Gain  Gain=Kp  SaturateOnIntegerOverflow=on  SampleTime=Ts  OutDataTypeStr=Inherit: Same as input  ParamDataTypeStr=Inherit: Same as input
  Kp5 : Gain  Gain=Ki  SaturateOnIntegerOverflow=on  SampleTime=Ts  OutDataTypeStr=Inherit: Same as input  ParamDataTypeStr=Inherit: Same as input
  Saturation2 : Saturate  UpperLimit=UpperLimit  LowerLimit=LowerLimit  SampleTime=Ts
  Sum6 : Sum  InputSameDT=on  SaturateOnIntegerOverflow=on  SampleTime=Ts  OutDataTypeStr=Inherit: Same as first input
  Zero-Order Hold : ZeroOrderHold  SampleTime=Ts
  Out : Outport  SampleTime=Ts  InitialOutput=0  VectorParamsAs1DForOutWhenUnconnected=off
  wires:
  Zero-Order Hold/1 -> Sum6/1
  Saturation2/1 -> Out/1
  Discrete-Time Integrator/1 -> Sum6/2
  Kp4/1 -> Zero-Order Hold/1
  Kp5/1 -> Discrete-Time Integrator/1
  Sum6/1 -> Saturation2/1
  Error/1 -> Kp5/1, Kp4/1

== system WindFarmType4AverageModel/Noble Ellenburg (81 MW)/Wind Farm/Control/Grid-side converter Control system/Discrete PI Controller ==
  note: Discrete PID Controller
  note: Pierre Giroux, Gilbert Sybille
      | Power System Simulation Laboratory
      | IREQ, Hydro-Quebc
  Error : Inport  SampleTime=Ts
  Discrete-Time Integrator : DiscreteIntegrator  InitialCondition=Init  SampleTime=Ts  LimitOutput=on  UpperSaturationLimit=UpperLimit  LowerSaturationLimit=LowerLimit  ICPrevOutput=DiscIntNeverNeededParam  ICPrevScaledInput=DiscIntNeverNeededParam
  Kp4 : Gain  Gain=Kp  SaturateOnIntegerOverflow=on  SampleTime=Ts  OutDataTypeStr=Inherit: Same as input  ParamDataTypeStr=Inherit: Same as input
  Kp5 : Gain  Gain=Ki  SaturateOnIntegerOverflow=on  SampleTime=Ts  OutDataTypeStr=Inherit: Same as input  ParamDataTypeStr=Inherit: Same as input
  Saturation2 : Saturate  UpperLimit=UpperLimit  LowerLimit=LowerLimit  SampleTime=Ts
  Sum6 : Sum  InputSameDT=on  SaturateOnIntegerOverflow=on  SampleTime=Ts  OutDataTypeStr=Inherit: Same as first input
  Zero-Order Hold : ZeroOrderHold  SampleTime=Ts
  Out : Outport  SampleTime=Ts  InitialOutput=0  VectorParamsAs1DForOutWhenUnconnected=off
  wires:
  Zero-Order Hold/1 -> Sum6/1
  Saturation2/1 -> Out/1
  Discrete-Time Integrator/1 -> Sum6/2
  Kp4/1 -> Zero-Order Hold/1
  Kp5/1 -> Discrete-Time Integrator/1
  Sum6/1 -> Saturation2/1
  Error/1 -> Kp5/1, Kp4/1

== system WindFarmType4AverageModel/Noble Ellenburg (81 MW)/Wind Farm/Control/Grid-side converter Control system/Discrete PI Controller1 ==
  note: Discrete PID Controller
  note: Pierre Giroux, Gilbert Sybille
      | Power System Simulation Laboratory
      | IREQ, Hydro-Quebc
  Error : Inport  SampleTime=Ts
  Discrete-Time Integrator : DiscreteIntegrator  InitialCondition=Init  SampleTime=Ts  LimitOutput=on  UpperSaturationLimit=UpperLimit  LowerSaturationLimit=LowerLimit  ICPrevOutput=DiscIntNeverNeededParam  ICPrevScaledInput=DiscIntNeverNeededParam
  Kp4 : Gain  Gain=Kp  SaturateOnIntegerOverflow=on  SampleTime=Ts  OutDataTypeStr=Inherit: Same as input  ParamDataTypeStr=Inherit: Same as input
  Kp5 : Gain  Gain=Ki  SaturateOnIntegerOverflow=on  SampleTime=Ts  OutDataTypeStr=Inherit: Same as input  ParamDataTypeStr=Inherit: Same as input
  Saturation2 : Saturate  UpperLimit=UpperLimit  LowerLimit=LowerLimit  SampleTime=Ts
  Sum6 : Sum  InputSameDT=on  SaturateOnIntegerOverflow=on  SampleTime=Ts  OutDataTypeStr=Inherit: Same as first input
  Zero-Order Hold : ZeroOrderHold  SampleTime=Ts
  Out : Outport  SampleTime=Ts  InitialOutput=0  VectorParamsAs1DForOutWhenUnconnected=off
  wires:
  Zero-Order Hold/1 -> Sum6/1
  Saturation2/1 -> Out/1
  Discrete-Time Integrator/1 -> Sum6/2
  Kp4/1 -> Zero-Order Hold/1
  Kp5/1 -> Discrete-Time Integrator/1
  Sum6/1 -> Saturation2/1
  Error/1 -> Kp5/1, Kp4/1

== system WindFarmType4AverageModel/Noble Ellenburg (81 MW)/Wind Farm/Control/Grid-side converter Control system/INT ==
  note: INTEGRATOR (Trapezoidal) with External limits & Reset & Hold
  Max : Inport
  Min : Inport  Port=2
  In : Inport  Port=3
  Ki : Inport  Port=4
  Hold : Inport  Port=5
  Reset : Inport  Port=6
  Reset Value : Inport  Port=7
  Gain : Gain  Gain=Ts* 0.5  SaturateOnIntegerOverflow=on  OutDataTypeStr=Inherit: Same as input  ParamDataTypeStr=Inherit: Same as input
  IC = 0 : UnitDelay  SampleTime=Ts  HasFrameUpgradeWarning=on
  IC = i_ic : UnitDelay  SampleTime=Ts  HasFrameUpgradeWarning=on
  Logical Operator4 : Logic  Operator=OR
  MinMax : MinMax  Inputs=2  InputSameDT=on  SaturateOnIntegerOverflow=on
  MinMax1 : MinMax  Function=max  Inputs=2  InputSameDT=on  SaturateOnIntegerOverflow=on
  Product : Product  SaturateOnIntegerOverflow=on  OutDataTypeStr=Inherit: Same as first input
  S6 : Subsystem  mask(Limiter with External Limits){}
      mask Display: disp('      Limiter\n')
  Sum : Sum  InputSameDT=on  SaturateOnIntegerOverflow=on  OutDataTypeStr=Inherit: Same as first input
  Sum1 : Sum  InputSameDT=on  SaturateOnIntegerOverflow=on  OutDataTypeStr=Inherit: Same as first input
  Switch2 : Switch  Threshold=0.5
  Switch3 : Switch  Threshold=0.5
  Switch7 : Switch  Threshold=0.5
  Out : Outport  InitialOutput=0  VectorParamsAs1DForOutWhenUnconnected=off
  wires:
  Switch7/1 -> Switch3/1, Sum/2, Switch2/1
  IC = i_ic/1 -> Switch7/3
  Min/1 -> MinMax1/2, Switch3/3
  Switch3/1 -> MinMax1/1
  MinMax1/1 -> S6/3(MIN)
  MinMax/1 -> S6/1(MAX)
  Reset Value/1 -> Switch7/1
  Max/1 -> MinMax/2, Switch2/3
  Switch2/1 -> MinMax/1
  Logical Operator4/1 -> Switch3/2, Switch2/2
  Reset/1 -> Logical Operator4/2, Switch7/2
  Hold/1 -> Logical Operator4/1
  Sum/1 -> S6/2(In)
  Product/1 -> Sum/1
  In/1 -> Sum1/1, IC = 0/1
  IC = 0/1 -> Sum1/2
  Ki/1 -> Gain/1
  Sum1/1 -> Product/2
  Gain/1 -> Product/1
  S6/1("  ") -> Out/1, IC = i_ic/1
